simulink model "GSMP"  (R2016b)
settings: Solver=VariableStepAuto  StartTime=0.0  StopTime=20  RelTol=1e-3
values from neighbouring files (symbols this model uses):
  A_lin = [ -R_GSM/L_GSM, 0, -k_GSM/L_GSM, 0;      0, 0, 1, -1;      k_GSM/J_GSM, -c_GSMP/J_GSM, -(d_GSMP + d_vGSM)/J_GSM, d_GSMP/J_GSM;      0, c_GSMP/J_P, d_GSMP/J_P, -(d_GSMP + d_vP + 2*d_qP*w_P_r)/J_P]    [aufgabe_4.m]    (also in aufgabe_6.m)
  A_red = [0,1,-1;  -c_GSMP/J_GSM, -(k_GSM^2/R_GSM + d_GSMP + d_vGSM)/J_GSM, d_GSMP/J_GSM;  c_GSMP/J_P, d_GSMP/J_P, -(d_GSMP + d_vP + 2*d_qP*w_P_r_red)/J_P]    [aufgabe_4.m]    (also in aufgabe_6.m)
  b_lin = [bu_lin bd_lin]    [aufgabe_4.m]    (also in aufgabe_6.m)
  b_red = [bu_red bd_red]    [aufgabe_4.m]    (also in aufgabe_6.m)
  M_ext_r = 0    [aufgabe_4.m]    (also in aufgabe_6.m)
  phi_GSMP_r = ((k_GSM^2 + R_GSM*d_vGSM)*(R_GSM*d_vP + R_GSM*d_vGSM -      (k_GSM^4 + R_GSM^2*d_vP^2 + R_GSM^2*d_vGSM^2 -      4*M_ext_r*R_GSM^2*d_qP - 4*R_GSM^2*d_cP*d_qP -      4*R_GSM^2*d_cGSM*d_qP + 2*R_GSM^2*d_vP*d_vGSM +      2*R_GSM*d_vP*k_GSM^2 + 2*R_GSM*d_vGSM*k_GSM^2 +      4*R_GSM*d_qP*k_GSM*u_GSM_r)^(1/2) + k_GSM^2))/(2*R_GSM^2*c_GSMP*d_qP)     - (R_GSM*d_cGSM - k_GSM*u_GSM_r)/(R_GSM*c_GSMP)    [aufgabe_4.m]    (also in aufgabe_6.m)
  u_GSM_r = 5.6    [aufgabe_4.m]    (also in aufgabe_6.m)
  w_GSM_r = -(R_GSM*d_vP + R_GSM*d_vGSM - (k_GSM^4 + R_GSM^2*d_vP^2 +      R_GSM^2*d_vGSM^2 - 4*M_ext_r*R_GSM^2*d_qP -      4*R_GSM^2*d_cP*d_qP - 4*R_GSM^2*d_cGSM*d_qP +      2*R_GSM^2*d_vP*d_vGSM + 2*R_GSM*d_vP*k_GSM^2 +      2*R_GSM*d_vGSM*k_GSM^2 + 4*R_GSM*d_qP*k_GSM*u_GSM_r)^(1/2) +      k_GSM^2)/(2*R_GSM*d_qP)    [aufgabe_4.m]    (also in aufgabe_6.m)
  w_P_r = -(R_GSM*d_vP + R_GSM*d_vGSM - (k_GSM^4 + R_GSM^2*d_vP^2 +      R_GSM^2*d_vGSM^2 - 4*M_ext_r*R_GSM^2*d_qP -      4*R_GSM^2*d_cP*d_qP - 4*R_GSM^2*d_cGSM*d_qP +      2*R_GSM^2*d_vP*d_vGSM + 2*R_GSM*d_vP*k_GSM^2 +      2*R_GSM*d_vGSM*k_GSM^2 + 4*R_GSM*d_qP*k_GSM*u_GSM_r)^(1/2) +      k_GSM^2)/(2*R_GSM*d_qP)    [aufgabe_4.m]    (also in aufgabe_5.m = -(R_GSM*d_vP + R_GSM*d_vGSM - (k_GSM^4 + R_GSM^2*d_vP^2 +   ; aufgabe_6.m)
undefined symbols (not defined in the file): c_GSMP, d_cGSM, d_cP, d_GSMP, d_qP, d_vGSM, d_vP, i_GSM_0, J_GSM, J_P, k_GSM, L_GSM, phi_GSMP_0, R_GSM, w_GSM_0, w_P_0
settings Model: Creator=M  LastModifiedBy=M

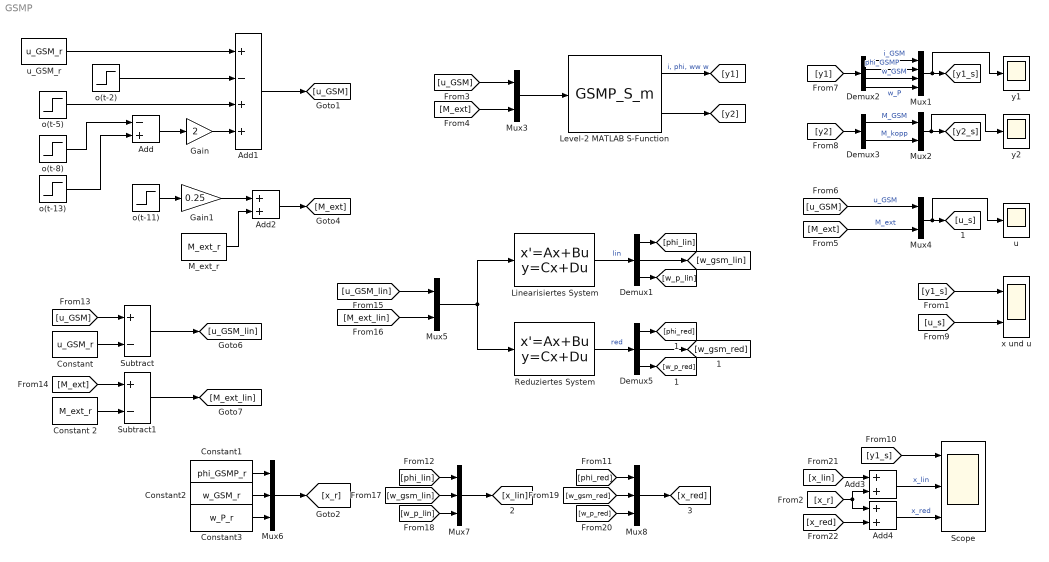
== system GSMP ==
  Add : Sum  Inputs=-+
  Add1 : Sum  Inputs=+-++
  Add2 : Sum
  Add3 : Sum
  Add4 : Sum
  Constant : Constant  Value=u_GSM_r
  Constant 2 : Constant  Value=M_ext_r
  Constant1 : Constant  Value=phi_GSMP_r
  Constant2 : Constant  Value=w_GSM_r
  Constant3 : Constant  Value=w_P_r
  Demux1 : Demux  Outputs=3
  Demux2 : Demux
  Demux3 : Demux  Outputs=2
  Demux5 : Demux  Outputs=3
  Gain : Gain  Gain=2
  Gain1 : Gain  Gain=0.25
  Level-2 MATLAB S-Function : M-S-Function  FunctionName=GSMP_S_m  Parameters=L_GSM, R_GSM, k_GSM, J_GSM, d_cGSM, d_vGSM, J_P, d_cP, d_vP, d_qP, c_GSMP, d_GSMP, i_GSM_0, phi_GSMP_0, w_GSM_0, w_P_0  mask{L_GSM=L_GSM, R_GSM=R_GSM, k_GSM=k_GSM, J_GSM=J_GSM, d_cGSM=d_cGSM, d_vGSM=d_vGSM, J_P=J_P, d_cP=d_cP, d_vP=d_vP, d_qP=d_qP, c_GSMP=c_GSMP, d_GSMP=d_GSMP, i_GSM_0=i_GSM_0, phi_GSMP_0=phi_GSMP_0, w_GSM_0=w_GSM_0, w_P_0=w_P_0}
      mask prompts: i_GSM_0 "i_GSM"; phi_GSMP_0 "phi_GSMP"; w_GSM_0 "w_GSM"; w_P_0 "w_P"
      mask DialogControl Container3 Prompt: Anfangszustände
  Linearisiertes System : StateSpace  A=A_lin  B=b_lin  C=[0 1 0 0; 0 0 1 0; 0 0 0 1]  D=[0 0; 0 0; 0 0]  X0=0
  M_ext_r : Constant  Value=M_ext_r
  Mux1 : Mux
  Mux{2..5} (4 alike) : Mux  Inputs=2
  Mux6 : Mux  Inputs=3
  Mux7 : Mux  Inputs=3
  Mux8 : Mux  Inputs=3
  Reduziertes System : StateSpace  A=A_red  B=b_red  C=[1 0 0; 0 1 0; 0 0 1]  D=[0 0; 0 0; 0 0]  X0=0
  Scope : Scope  NumInputPorts=3
  Subtract : Sum  Inputs=+-
  Subtract1 : Sum  Inputs=+-
  o(t-11) : Step  Time=11  SampleTime=0
  o(t-13) : Step  Time=13  SampleTime=0
  o(t-2) : Step  Time=2  SampleTime=0
  o(t-5) : Step  Time=5  SampleTime=0
  o(t-8) : Step  Time=8  SampleTime=0
  u : Scope
  "u_GSM_r " : Constant  Value=u_GSM_r
  x und u : Scope  NumInputPorts=2
  "y1 " : Scope
  "y2 " : Scope
  wires:
  Mux3/1 -> Level-2 MATLAB S-Function/1
  [u_GSM] -> Mux3/1
  [M_ext] -> Mux3/2
  Level-2 MATLAB S-Function/1 -> [y1]  "i, phi, ww w"
  Level-2 MATLAB S-Function/2 -> [y2]
  "u_GSM_r "/1 -> Add1/1
  Add1/1 -> [u_GSM]
  o(t-2)/1 -> Add1/2
  o(t-8)/1 -> Add/1
  o(t-13)/1 -> Add/2
  Add/1 -> Gain/1
  o(t-5)/1 -> Add1/3
  Gain/1 -> Add1/4
  Gain1/1 -> Add2/1
  M_ext_r/1 -> Add2/2
  o(t-11)/1 -> Gain1/1
  Add2/1 -> [M_ext]
  [y1] -> Demux2/1
  Demux2/1 -> Mux1/1  "i_GSM"
  Demux2/2 -> Mux1/2  "phi_GSMP"
  Demux2/3 -> Mux1/3  "w_GSM"
  Demux2/4 -> Mux1/4  "w_P"
  Mux1/1 -> "y1 "/1, [y1_s]
  Demux3/2 -> Mux2/2  "M_kopp"
  [y2] -> Demux3/1
  Demux3/1 -> Mux2/1  "M_GSM"
  Mux2/1 -> "y2 "/1, [y2_s]
  [u_GSM] -> Mux4/1  "u_GSM"
  [M_ext] -> Mux4/2  "M_ext"
  Mux4/1 -> u/1, [u_s]
  [y1_s] -> x und u/1
  [u_s] -> x und u/2
  Mux5/1 -> Reduziertes System/1, Linearisiertes System/1
  Subtract/1 -> [u_GSM_lin]
  Constant/1 -> Subtract/2
  [u_GSM] -> Subtract/1
  Subtract1/1 -> [M_ext_lin]
  Constant 2/1 -> Subtract1/2
  [M_ext] -> Subtract1/1
  [M_ext_lin] -> Mux5/2
  [u_GSM_lin] -> Mux5/1
  Linearisiertes System/1 -> Demux1/1  "lin"
  Demux1/1 -> [phi_lin]
  Demux1/2 -> [w_gsm_lin]
  Demux1/3 -> [w_p_lin]
  Reduziertes System/1 -> Demux5/1  "red"
  Demux5/1 -> [phi_red]
  Demux5/3 -> [w_p_red]
  Constant2/1 -> Mux6/2
  Constant1/1 -> Mux6/1
  Constant3/1 -> Mux6/3
  Mux6/1 -> [x_r]
  [x_r] -> Add3/2, Add4/1
  Add3/1 -> Scope/2  "x_lin"
  Add4/1 -> Scope/3  "x_red"
  [y1_s] -> Scope/1
  [phi_lin] -> Mux7/1
  [w_gsm_lin] -> Mux7/2
  [w_p_lin] -> Mux7/3
  [phi_red] -> Mux8/1
  [w_gsm_red] -> Mux8/2
  [w_p_red] -> Mux8/3
  Mux7/1 -> [x_lin]
  Mux8/1 -> [x_red]
  [x_lin] -> Add3/1
  [x_red] -> Add4/2
  Demux5/2 -> [w_gsm_red]
